simulink model "Vehicle_Plant_Model"  (R2016b)
settings: Solver=ode3  StartTime=0.0  StopTime=120  FixedStep=0.01  RelTol=1e-3  EnableMultiTasking=on
model workspace (MAT data in the model file):
  A = Simulink.Parameter
  A.Value = 2.4
  A.DataType = 'auto'
  A.Dimensions = [1 1]
  Cd = Simulink.Parameter
  Cd.Value = 0.32
  Cd.DataType = 'auto'
  Cd.Dimensions = [1 1]
  Cr = Simulink.Parameter
  Cr.Value = 0.01
  Cr.DataType = 'auto'
  Cr.Dimensions = [1 1]
  Tm = Simulink.Parameter
  Tm.Value = 190
  Tm.DataType = 'auto'
  Tm.Dimensions = [1 1]
  betac = Simulink.Parameter
  betac.Value = 0.4
  betac.DataType = 'auto'
  betac.Dimensions = [1 1]
  g = Simulink.Parameter
  g.Value = 9.8
  g.DataType = 'auto'
  g.Dimensions = [1 1]
  m = Simulink.Parameter
  m.Value = 1000
  m.DataType = 'auto'
  m.Dimensions = [1 1]
  omegam = Simulink.Parameter
  omegam.Value = 420
  omegam.DataType = 'auto'
  omegam.Dimensions = [1 1]
  rho = Simulink.Parameter
  rho.Value = 1.2
  rho.DataType = 'auto'
  rho.Dimensions = [1 1]
libraries: simulink_extras x1
settings Model: Creator=root  LastModifiedBy=Atef
settings SolverCC: ShapePreserveControl=EnableAll
settings DataIOCC: ReturnWorkspaceOutputs=on
settings OptimizationCC: DefaultUnderspecifiedDataType=single  EfficientFloat2IntCast=on  LifeSpan=inf
settings DebuggingCC: SFUnexpectedBacktrackingDiag=warning  SFNoUnconditionalDefaultTransitionDiag=warning  SFExecutionAtInitializationDiag=none
settings HardwareCC: ProdBitPerSizeT=32  ProdBitPerPtrDiffT=32  ProdWordSize=32  ProdHWDeviceType=Specified
settings ModelReferenceCC: PropagateSignalLabelsOutOfModel=off
settings GRTTargetCC: TargetLangStandard=C89/C90 (ANSI)  GeneratePreprocessorConditionals=Disable all
settings ConfigComp: CovMetricSettings=dw  CovHtmlReporting=on  CovSaveCumulativeToWorkspaceVar=on  CovSaveSingleToWorkspaceVar=on  CovExternalEMLEnable=off
settings ConfigurationSet: Description=SimMechanics 2G

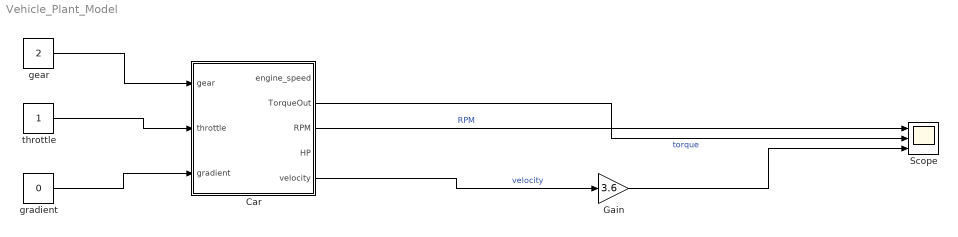
== system Vehicle_Plant_Model ==
  Car : Subsystem
  Gain : Gain  Gain=3.6
  Scope : Scope  NumInputPorts=3
  gear : Constant  Value=2
  gradient : Constant  Value=0
  throttle : Constant
  wires:
  Car/5(velocity) -> Gain/1  "velocity"
  Car/3(RPM) -> Scope/1  "RPM"
  Gain/1 -> Scope/3
  throttle/1 -> Car/2(throttle)
  gear/1 -> Car/1(gear)
  gradient/1 -> Car/3(gradient)
  Car/2(TorqueOut) -> Scope/2  "torque"

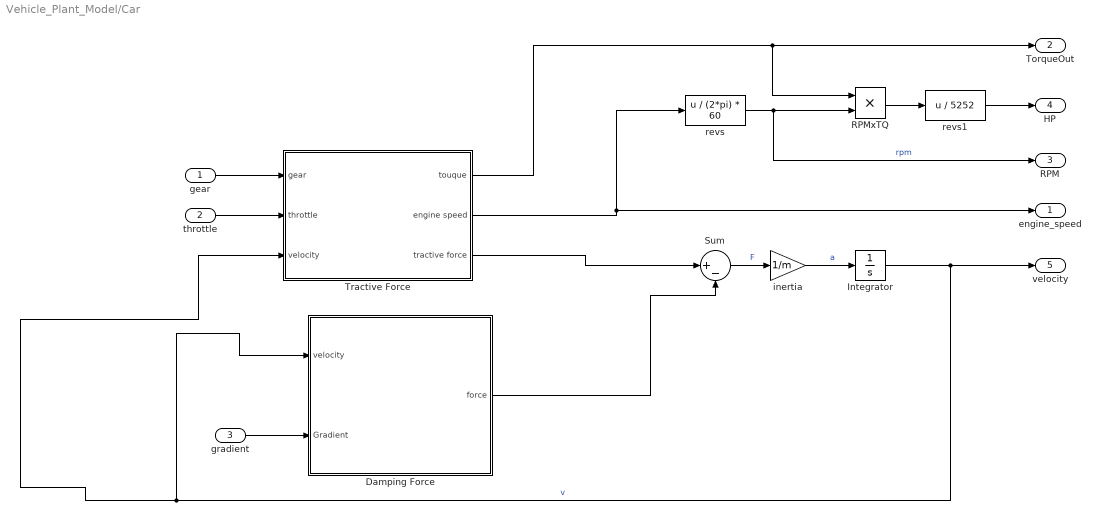
== system Vehicle_Plant_Model/Car ==
  gear : Inport
  throttle : Inport  Port=2  OutMin=0  OutMax=1
  gradient : Inport  Port=3
  Damping Force : Subsystem
  Integrator : Integrator
  RPMxTQ : Product
  Sum : Sum  Inputs=|+-
  Tractive Force : Subsystem
  inertia : Gain  Gain=1/m
  revs : Fcn  Expr=u / (2*pi) * 60
  revs1 : Fcn  Expr=u / 5252
  engine_speed : Outport
  TorqueOut : Outport  Port=2
  RPM : Outport  Port=3
  HP : Outport  Port=4
  velocity : Outport  Port=5
  wires:
  inertia/1 -> Integrator/1  "a"
  Sum/1 -> inertia/1  "F"
  Integrator/1 -> Tractive Force/3(velocity), Damping Force/1(velocity), velocity/1  "v"
  revs/1 -> RPM/1, RPMxTQ/2  "rpm"
  RPMxTQ/1 -> revs1/1
  revs1/1 -> HP/1
  Tractive Force/2(engine speed) -> revs/1, engine_speed/1
  Tractive Force/1(touque) -> TorqueOut/1, RPMxTQ/1
  gear/1 -> Tractive Force/1(gear)
  throttle/1 -> Tractive Force/2(throttle)
  Tractive Force/3(tractive force) -> Sum/1
  gradient/1 -> Damping Force/2(Gradient)
  Damping Force/1(force) -> Sum/2

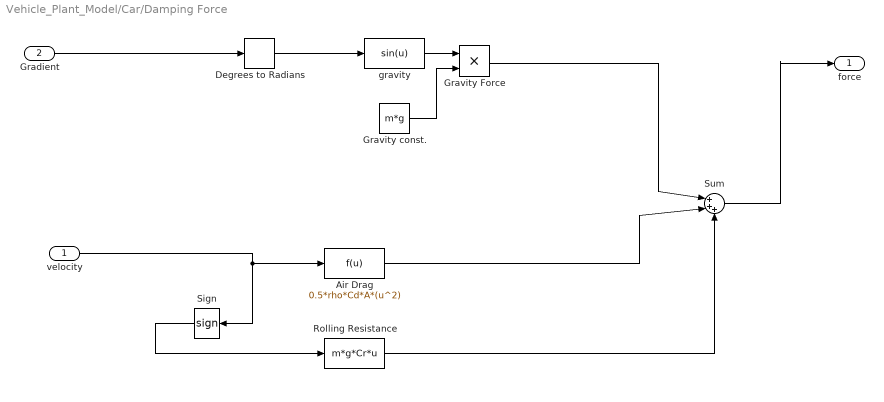
== system Vehicle_Plant_Model/Car/Damping Force ==
  velocity : Inport
  Gradient : Inport  Port=2
  Air Drag : Fcn  Expr=0.5*rho*Cd*A*(u^2)
  Degrees to Radians : simulink_extras/Transformations/Degrees to Radians
  Gravity Force : Product
  Gravity const. : Constant  Value=m*g
  Rolling Resistance : Fcn  Expr=m*g*Cr*u
  Sign : Signum
  Sum : Sum  Inputs=|+++
  gravity : Fcn  Expr=sin(u)
  force : Outport
  wires:
  Sign/1 -> Rolling Resistance/1
  Rolling Resistance/1 -> Sum/3
  Gravity const./1 -> Gravity Force/2
  Gradient/1 -> Degrees to Radians/1
  Degrees to Radians/1 -> gravity/1
  gravity/1 -> Gravity Force/1
  Air Drag/1 -> Sum/2
  Gravity Force/1 -> Sum/1
  velocity/1 -> Air Drag/1, Sign/1
  Sum/1 -> force/1

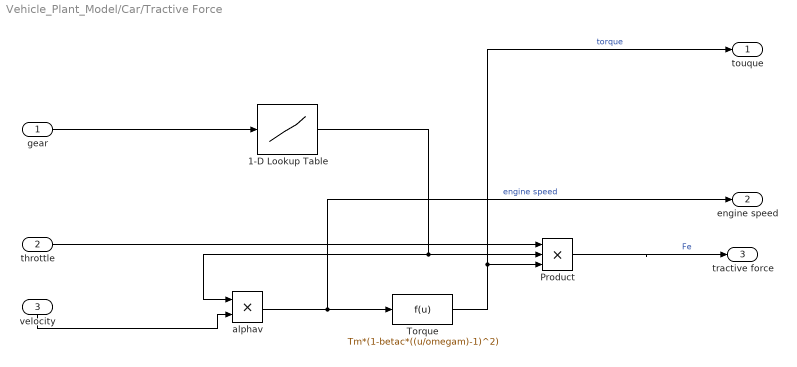
== system Vehicle_Plant_Model/Car/Tractive Force ==
  gear : Inport
  throttle : Inport  Port=2
  velocity : Inport  Port=3
  1-D Lookup Table : Lookup_n-D  NumberOfTableDimensions=1  BreakpointsForDimension1=int16([1,2,3,4,5]);  Table=int16([40,25,16,12,10]);  InternalRulePriority=Speed  RndMeth=Simplest  InputSameDT=on
  Product : Product  Inputs=3
  Torque : Fcn  Expr=Tm*(1-betac*((u/omegam)-1)^2)
  alphav : Product
  touque : Outport
  engine speed : Outport  Port=2
  tractive force : Outport  Port=3
  wires:
  gear/1 -> 1-D Lookup Table/1
  Torque/1 -> touque/1, Product/3  "torque"
  throttle/1 -> Product/1
  1-D Lookup Table/1 -> Product/2, alphav/1
  alphav/1 -> engine speed/1, Torque/1  "engine speed"
  Product/1 -> tractive force/1  "Fe"
  velocity/1 -> alphav/2
